simulink model "controle_PI"  (R2015a)
settings: Solver=ode1  SolverMode=SingleTasking  StartTime=0.0  StopTime=10.0  FixedStep=0.01  RelTol=1e-3
values from neighbouring files (symbols this model uses):
  KNL = 59.7881    [exp11.m]
  Kp = 1.604    [exp11.m]
  Kpi = 0.5    [exp11.m]
  Kt = KtL    (= 0.0169213973799)    [exp11.m]
  T = 0.27    [exp11.m]
undefined symbols (not defined in the file): phi
settings Model: CovSFcnEnable=off  Creator=rpm  LastModifiedBy=sasuk
settings DataIOCC: LimitDataPoints=off  SignalLoggingSaveFormat=ModelDataLogs  SaveOutput=off  SignalLogging=off  TimeSaveName=t
settings OptimizationCC: ExpressionDepthLimit=2147483647  InitFltsAndDblsToZero=on
settings DebuggingCC: UnderspecifiedInitializationDetection=Classic  MergeDetectMultiDrivingBlocksExec=none  FcnCallInpInsideContextMsg=UseLocalSettings  StateNameClashWarn=warning
settings GRTTargetCC: CombineOutputUpdateFcns=off  GRTInterface=on

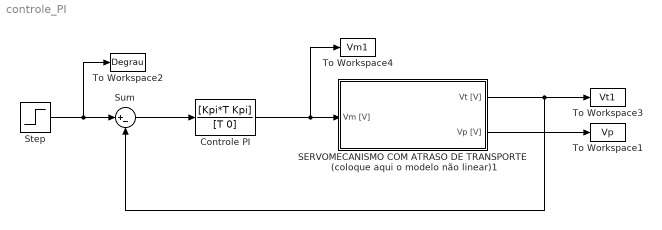
== system controle_PI ==
  Controle PI : TransferFcn  Numerator=[Kpi*T Kpi]  Denominator=[T 0]
  SERVOMECANISMO COM ATRASO DE TRANSPORTE (coloque aqui o modelo não linear)1 : Subsystem
  Step : Step  Time=0  After=1.59  SampleTime=0
  Sum : Sum  Inputs=|+-
  To Workspace1 : ToWorkspace  VariableName=Vp  SampleTime=-1
  To Workspace2 : ToWorkspace  VariableName=Degrau  SampleTime=-1
  To Workspace3 : ToWorkspace  VariableName=Vt1  SampleTime=-1
  To Workspace4 : ToWorkspace  VariableName=Vm1  SampleTime=-1
  wires:
  SERVOMECANISMO COM ATRASO DE TRANSPORTE (coloque aqui o modelo não linear)1/1(Vt [V]) -> Sum/2, To Workspace3/1
  Controle PI/1 -> SERVOMECANISMO COM ATRASO DE TRANSPORTE (coloque aqui o modelo não linear)1/1(Vm [V]), To Workspace4/1
  Sum/1 -> Controle PI/1
  Step/1 -> To Workspace2/1, Sum/1
  SERVOMECANISMO COM ATRASO DE TRANSPORTE (coloque aqui o modelo não linear)1/2(Vp [V]) -> To Workspace1/1

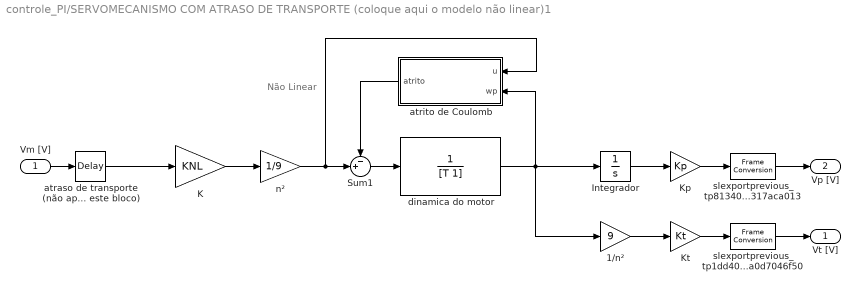
== system controle_PI/SERVOMECANISMO COM ATRASO DE TRANSPORTE (coloque aqui o modelo não linear)1 ==
  note: Não
      | Linear
  Vm [V] : Inport
  1/n² : Gain  Gain=9
  Integrador : Integrator
  K : Gain  Gain=KNL
  Kp : Gain  Gain=Kp
  Kt : Gain  Gain=Kt
  Sum1 : Sum  Inputs=-+|
  atraso de transporte (não apague este bloco) : TransportDelay  DelayTime=0.3
  atrito de Coulomb : Subsystem  mask{phi=phi}
      mask Display: fprintf('phi = %3.1f', phi)
  dinamica do motor : TransferFcn  Denominator=[T 1]
  n² : Gain  Gain=1/9
  slexportprevious_tp1dd40cb0_336a_46da_8b79_bfa0d7046f50 : FrameConversion  OutFrame=Sample-based
  slexportprevious_tp8134031d_9c58_445d_bef1_a0d317aca013 : FrameConversion  OutFrame=Sample-based
  Vt [V] : Outport
  Vp [V] : Outport  Port=2
  wires:
  Vm [V]/1 -> atraso de transporte (não apague este bloco)/1
  dinamica do motor/1 -> 1/n²/1, Integrador/1, atrito de Coulomb/2(wp)
  Integrador/1 -> Kp/1
  K/1 -> n²/1
  n²/1 -> atrito de Coulomb/1(u), Sum1/2
  atrito de Coulomb/1(atrito) -> Sum1/1
  Sum1/1 -> dinamica do motor/1
  1/n²/1 -> Kt/1
  Kp/1 -> slexportprevious_tp8134031d_9c58_445d_bef1_a0d317aca013/1
  Kt/1 -> slexportprevious_tp1dd40cb0_336a_46da_8b79_bfa0d7046f50/1
  atraso de transporte (não apague este bloco)/1 -> K/1
  slexportprevious_tp1dd40cb0_336a_46da_8b79_bfa0d7046f50/1 -> Vt [V]/1
  slexportprevious_tp8134031d_9c58_445d_bef1_a0d317aca013/1 -> Vp [V]/1

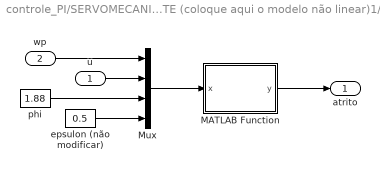
== system controle_PI/SERVOMECANISMO COM ATRASO DE TRANSPORTE (coloque aqui o modelo não linear)1/atrito de Coulomb ==
  u : Inport
  wp : Inport  Port=2
  MATLAB Function : MATLAB Function  TreatAsAtomicUnit=on
  Mux : Mux
  epsulon (não modificar) : Constant  Value=0.5
  phi : Constant  Value=1.88
  atrito : Outport
  wires:
  u/1 -> Mux/2
  phi/1 -> Mux/3
  MATLAB Function/1(y) -> atrito/1
  wp/1 -> Mux/1
  epsulon (não modificar)/1 -> Mux/4
  Mux/1 -> MATLAB Function/1(x)

== matlab function controle_PI/SERVOMECANISMO COM ATRASO DE TRANSPORTE (coloque aqui o modelo não linear)1/atrito de Coulomb/MATLAB Function ==
  data: x input size=4; y output size=1
function y = nl_coulomb(x)
% Atrito de Coulomb
% Para uso de nl_template.mdl

wp  = x(1); 
u   = x(2); 
phi = x(3); 
epsulon = x(4);

y = 0;

if wp > epsulon
    y = phi;
elseif wp < -epsulon
    y = -phi;
elseif wp >= 0
    y = min(phi,abs(u));
elseif wp < 0
    y = max(-phi,-abs(u));
end
